simulink library "LinSysLib"  (R2018b)
settings: Solver=VariableStepAuto  StartTime=0.0  StopTime=10.0  RelTol=1e-3
values from neighbouring files (symbols this model uses):
  A = [-b/J, Kt/J; -Ke/l, -r/l]    [makedcmotorparams.m]    (also in tanks.m = [-1/Ti(1, Area(1))            0;      Area(1)/Area(2)/Ti(h0,)
  B = [0; 1/l]    [makedcmotorparams.m]    (also in tanks.m = [1/Area(1); 0])
  C = [1, 1]    [makedcmotorparams.m]    (also in tanks.m = [0 1])
  K = place(Ad, Bd, cpoles)    [makedcmotorparams.m]
  L = place(Ad', Cd', [0.6, 0]).'    [makedcmotorparams.m]    (also in tanks.m = place(A', C', [-100 -2])')
  r = 32.91    [makedcmotorparams.m]
  T = connect(ctrl, sys, obsv, sum_ref, 'xref', 'x1')    [makedcmotorparams.m]
  x0 = zeros(2,1)    [makedcmotorparams.m]
undefined symbols (not defined in the file or in its folder): D, F, H, hatx0, z0
settings Model: Creator=ab1416  LastModifiedBy=ab1416

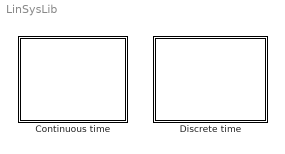
== system LinSysLib ==
  Continuous time : Subsystem
  Discrete time : Subsystem

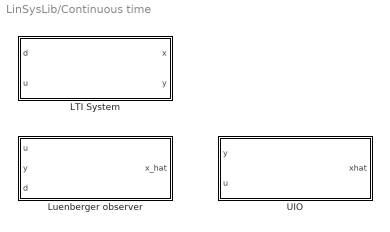
== system LinSysLib/Continuous time ==
  LTI System : Subsystem  mask{A=A, B=B, C=C, D=D, x0=x0}
      mask prompts: A "Matrix A:"; B "Matrix B:"; C "Matrix C:"; D "Matrix D:"; x0 "Initial condition:"
      mask help: State space model of an LTI system, with accessible state
      mask Display: disp('CT LTI System')
  Luenberger observer : Subsystem  mask{A=A, B=B, C=C, D=D, x0=hatx0, L=L}
      mask prompts: A "Matrix A"; B "Matrix B"; C "Matrix C"; D "Matrix D"; x0 "Initial conditions"; L "Gain"
      mask help: Continuous-Time Luenberger observer
      mask DialogControl Container5 Prompt: Reference Model
      mask DialogControl Container6 Prompt: Observer Parameters
      mask Display: disp('Luenberger\nObserver');
  UIO : Subsystem  mask{F_uio=F, H_uio=H, K_uio=K, B=B, T_uio=T, hatx0=z0}
      mask prompts: F_uio "F"; H_uio "H"; K_uio "K"; T_uio "T"; hatx0 "Initial condition"
      mask DialogControl Container3 Prompt: UIO design parameters
      mask Display: disp('UIO');

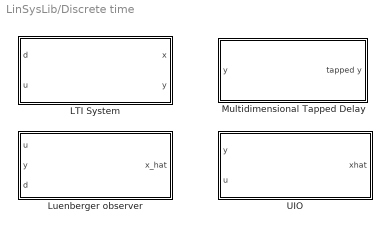
== system LinSysLib/Discrete time ==
  LTI System : Subsystem  mask{A=A, B=B, C=C, D=D, x0=x0}
      mask prompts: A "Matrix A:"; B "Matrix B:"; C "Matrix C:"; D "Matrix D:"; x0 "Initial condition:"
      mask help: State space model of an LTI system, with accessible state
      mask Display: disp('DT LTI System')
  Luenberger observer : Subsystem  mask{A=A, B=B, C=C, D=D, hatx0=hatx0, L=L}
      mask prompts: A "Matrix A"; B "Matrix B"; C "Matrix C"; D "Matrix D"; hatx0 "Initial conditions"; L "Gain"
      mask help: Continuous-Time Luenberger observer
      mask DialogControl Container5 Prompt: Reference Model
      mask DialogControl Container6 Prompt: Observer Parameters
      mask Display: disp('Discrete\nLuenberger\nObserver');
  Multidimensional Tapped Delay : Subsystem  mask{r=r}
      mask prompts: r "Delays"
      mask TypeOptions r: MATLAB Function1/r
  UIO : Subsystem  mask{F_uio=F, H_uio=H, K_uio=K, B=B, T_uio=T, hatx0=z0}
      mask prompts: F_uio "F"; H_uio "H"; K_uio "K"; T_uio "T"; hatx0 "Initial condition"
      mask DialogControl Container3 Prompt: UIO design parameters
      mask Display: disp(' Discrete\nUIO');

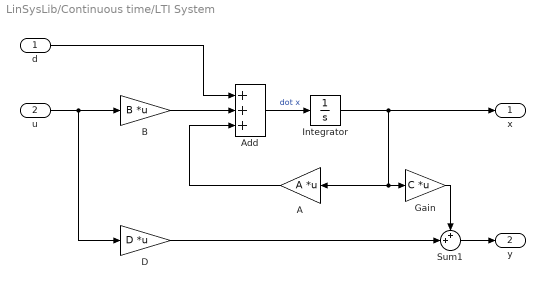
== system LinSysLib/Continuous time/LTI System ==
  d : Inport
  u : Inport  Port=2  PortDimensions=size(B,2)
  A : Gain  Gain=A  Multiplication=Matrix(K*u)
  Add : Sum  Inputs=+++
  B : Gain  Gain=B  Multiplication=Matrix(K*u)
  D : Gain  Gain=D  Multiplication=Matrix(K*u)
  Gain : Gain  Gain=C  Multiplication=Matrix(K*u)
  Integrator : Integrator  InitialCondition=x0
  Sum1 : Sum  Inputs=++|
  x : Outport  PortDimensions=size(A,1)
  y : Outport  Port=2  PortDimensions=size(C,1)
  wires:
  d/1 -> Add/1
  Gain/1 -> Sum1/1
  D/1 -> Sum1/2
  Sum1/1 -> y/1
  A/1 -> Add/3
  Add/1 -> Integrator/1  "dot x"
  Integrator/1 -> Gain/1, A/1, x/1
  B/1 -> Add/2
  u/1 -> B/1, D/1

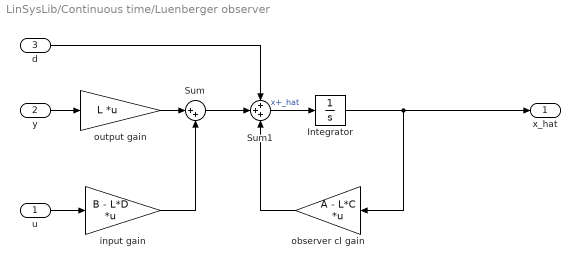
== system LinSysLib/Continuous time/Luenberger observer ==
  u : Inport
  y : Inport  Port=2
  d : Inport  Port=3
  Integrator : Integrator  InitialCondition=hatx0
  Sum : Sum  Inputs=|++
  Sum1 : Sum  Inputs=+++
  input gain : Gain  Gain=B - L*D  Multiplication=Matrix(K*u)
  observer cl gain : Gain  Gain=A - L*C  Multiplication=Matrix(K*u)
  output gain : Gain  Gain=L  Multiplication=Matrix(K*u)
  x_hat : Outport
  wires:
  u/1 -> input gain/1
  observer cl gain/1 -> Sum1/3
  input gain/1 -> Sum/2
  Sum1/1 -> Integrator/1  "x+_hat"
  y/1 -> output gain/1
  Integrator/1 -> observer cl gain/1, x_hat/1
  output gain/1 -> Sum/1
  Sum/1 -> Sum1/2
  d/1 -> Sum1/1

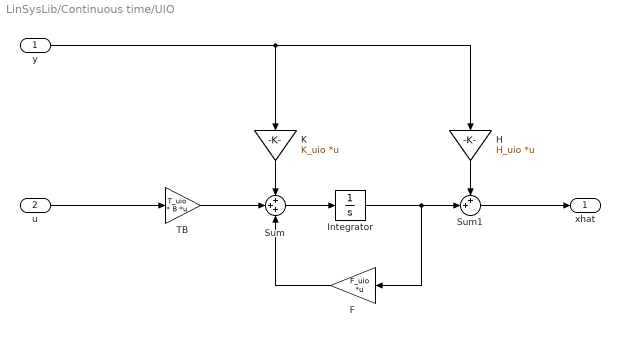
== system LinSysLib/Continuous time/UIO ==
  y : Inport
  u : Inport  Port=2
  F : Gain  Gain=F_uio  Multiplication=Matrix(K*u)
  H : Gain  Gain=H_uio  Multiplication=Matrix(K*u)
  Integrator : Integrator  InitialCondition=hatx0
  K : Gain  Gain=K_uio  Multiplication=Matrix(K*u)
  Sum : Sum  Inputs=+++
  Sum1 : Sum  Inputs=++|
  TB : Gain  Gain=T_uio * B  Multiplication=Matrix(K*u)
  xhat : Outport
  wires:
  u/1 -> TB/1
  TB/1 -> Sum/2
  y/1 -> H/1, K/1
  K/1 -> Sum/1
  Sum/1 -> Integrator/1
  Integrator/1 -> Sum1/2, F/1
  F/1 -> Sum/3
  H/1 -> Sum1/1
  Sum1/1 -> xhat/1

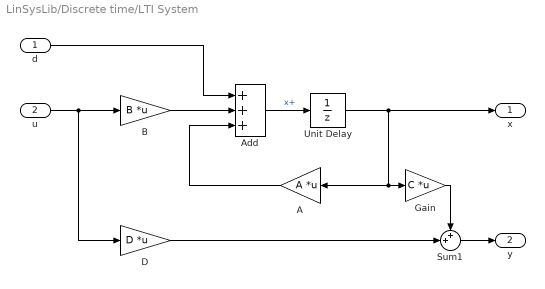
== system LinSysLib/Discrete time/LTI System ==
  d : Inport
  u : Inport  Port=2  PortDimensions=size(B,2)
  A : Gain  Gain=A  Multiplication=Matrix(K*u)
  Add : Sum  Inputs=+++
  B : Gain  Gain=B  Multiplication=Matrix(K*u)
  D : Gain  Gain=D  Multiplication=Matrix(K*u)
  Gain : Gain  Gain=C  Multiplication=Matrix(K*u)
  Sum1 : Sum  Inputs=++|
  Unit Delay : UnitDelay  InitialCondition=x0  SampleTime=-1
  x : Outport  PortDimensions=size(A,1)
  y : Outport  Port=2  PortDimensions=size(C,1)
  wires:
  u/1 -> D/1, B/1
  B/1 -> Add/2
  Unit Delay/1 -> x/1, A/1, Gain/1
  Add/1 -> Unit Delay/1  "x+"
  A/1 -> Add/3
  Sum1/1 -> y/1
  D/1 -> Sum1/2
  Gain/1 -> Sum1/1
  d/1 -> Add/1

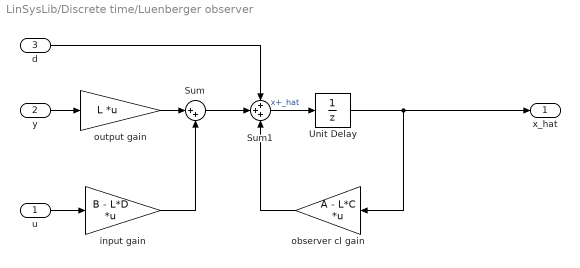
== system LinSysLib/Discrete time/Luenberger observer ==
  u : Inport
  y : Inport  Port=2
  d : Inport  Port=3
  Sum : Sum  Inputs=|++
  Sum1 : Sum  Inputs=+++
  Unit Delay : UnitDelay  InitialCondition=hatx0  SampleTime=-1
  input gain : Gain  Gain=B - L*D  Multiplication=Matrix(K*u)
  observer cl gain : Gain  Gain=A - L*C  Multiplication=Matrix(K*u)
  output gain : Gain  Gain=L  Multiplication=Matrix(K*u)
  x_hat : Outport
  wires:
  u/1 -> input gain/1
  observer cl gain/1 -> Sum1/3
  input gain/1 -> Sum/2
  Sum1/1 -> Unit Delay/1  "x+_hat"
  y/1 -> output gain/1
  Unit Delay/1 -> observer cl gain/1, x_hat/1
  output gain/1 -> Sum/1
  Sum/1 -> Sum1/2
  d/1 -> Sum1/1

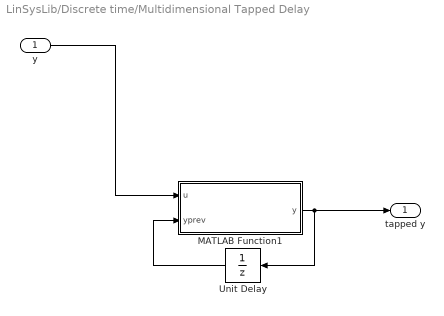
== system LinSysLib/Discrete time/Multidimensional Tapped Delay ==
  y : Inport
  MATLAB Function1 : MATLAB Function  TreatAsAtomicUnit=on  mask{r=r}
      mask prompts: r "Delays"
  Unit Delay : UnitDelay  SampleTime=-1
  tapped y : Outport
  wires:
  MATLAB Function1/1(y) -> Unit Delay/1, tapped y/1
  Unit Delay/1 -> MATLAB Function1/2(yprev)
  y/1 -> MATLAB Function1/1(u)

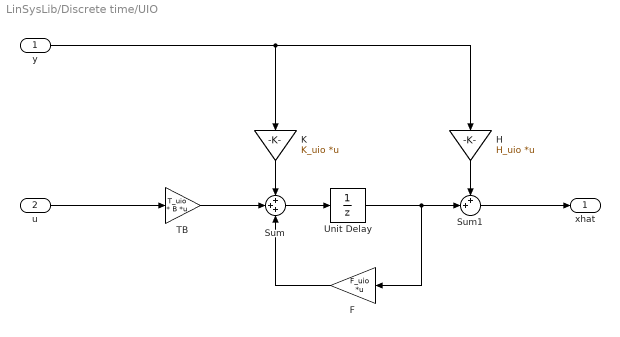
== system LinSysLib/Discrete time/UIO ==
  y : Inport
  u : Inport  Port=2
  F : Gain  Gain=F_uio  Multiplication=Matrix(K*u)
  H : Gain  Gain=H_uio  Multiplication=Matrix(K*u)
  K : Gain  Gain=K_uio  Multiplication=Matrix(K*u)
  Sum : Sum  Inputs=+++
  Sum1 : Sum  Inputs=++|
  TB : Gain  Gain=T_uio * B  Multiplication=Matrix(K*u)
  Unit Delay : UnitDelay  InitialCondition=hatx0  SampleTime=-1
  xhat : Outport
  wires:
  Sum1/1 -> xhat/1
  H/1 -> Sum1/1
  F/1 -> Sum/3
  Unit Delay/1 -> F/1, Sum1/2
  Sum/1 -> Unit Delay/1
  K/1 -> Sum/1
  y/1 -> K/1, H/1
  TB/1 -> Sum/2
  u/1 -> TB/1

== matlab function LinSysLib/Discrete time/Multidimensional Tapped Delay/MATLAB Function1 ==
  data: u input; y output; yprev input; r parameter
function y = tapDelay(u, yprev, r)

p = size(u,1);
y = zeros(p*r, size(u,2));

y(1:end-p, :) = yprev(p+1:end,:);
y(end-p+1:end,:) = u;

end
